simulink model "planta_PID_velocity"  (R2019b)
settings: Solver=ode23t  StartTime=0.0  StopTime=7  MaxStep=T  RelTol=1e-3  EnableMultiTasking=on
undefined symbols (not defined in the file): T
settings Model: Creator=fernandopassold  LastModifiedBy=fernandopassold
settings DataIOCC: LimitDataPoints=on  SaveFormat=Array  ReturnWorkspaceOutputs=off
settings OptimizationCC: LifeSpan=inf
settings DebuggingCC: SFUnexpectedBacktrackingDiag=warning  SFNoUnconditionalDefaultTransitionDiag=warning  SFExecutionAtInitializationDiag=none  ArithmeticOperatorsInVariantConditions=warning
settings HardwareCC: ProdBitPerPointer=32  ProdBitPerSizeT=32  ProdBitPerPtrDiffT=32  ProdLargestAtomicFloat=None  ProdIntDivRoundTo=Undefined  ProdEndianess=Unspecified  ProdWordSize=32  ProdHWDeviceType=32-bit Generic
settings ModelReferenceCC: PropagateSignalLabelsOutOfModel=off
settings SFSimCC: SimUseLocalCustomCode=off  CustomCodeUndefinedFunction=UseInterfaceOnly
settings RTWCC: RTWUseLocalCustomCode=off
settings CodeAppCC: StateflowObjectComments=on
settings GRTTargetCC: TargetLangStandard=C89/C90 (ANSI)  GeneratePreprocessorConditionals=Disable all
settings ConfigComp: CovMetricSettings=dw  CovHtmlReporting=on  CovSaveCumulativeToWorkspaceVar=on  CovSaveSingleToWorkspaceVar=on  CovExternalEMLEnable=off

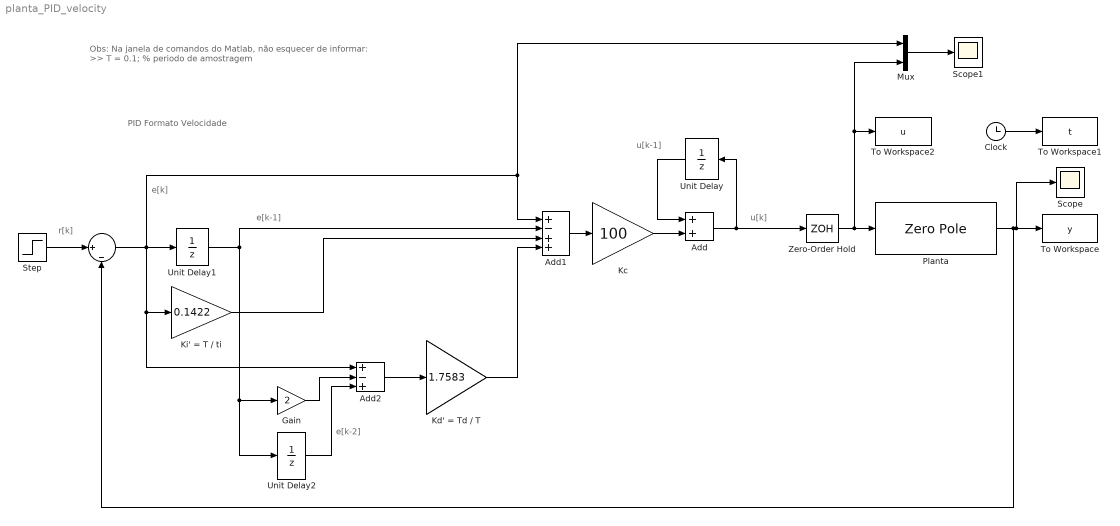
== system planta_PID_velocity ==
  note: Obs:
      | Na janela de comandos do Matlab, não esquecer de informar:
      | >> T = 0.1; % periodo de amostragem
  note: PID Formato Velocidade
  note: u[k-1]
  note: e[k-2]
  note: e[k-1]
  note: u[k]
  note: r[k]
  note: e[k]
  " " : Sum  Inputs=||+|-
  Add : Sum
  Add1 : Sum  Inputs=+|-|+|+
  Add2 : Sum  Inputs=+|-|+
  Clock : Clock
  Gain : Gain  Gain=2
  Kc : Gain  Gain=100
  Kd' = Td / T : Gain  Gain=1.7583
  Ki' = T / ti : Gain  Gain=0.1422
  Mux : Mux  Inputs=2
  Planta : ZeroPole  Zeros=[ ]  Poles="[-1  -2   -10]"
  Scope : Scope
  Scope1 : Scope
  Step : Step  Time=0  SampleTime=0
  To Workspace : ToWorkspace  VariableName=y  SaveFormat=Timeseries  SampleTime=-1
  To Workspace1 : ToWorkspace  VariableName=t  SampleTime=-1
  To Workspace2 : ToWorkspace  VariableName=u  SaveFormat=Timeseries  SampleTime=T
  Unit Delay : UnitDelay  SampleTime=T  HasFrameUpgradeWarning=on
  Unit Delay1 : UnitDelay  SampleTime=T  HasFrameUpgradeWarning=on
  Unit Delay2 : UnitDelay  SampleTime=T  HasFrameUpgradeWarning=on
  Zero-Order Hold : ZeroOrderHold  SampleTime=T
  wires:
  Step/1 -> " "/1
  Zero-Order Hold/1 -> Mux/2, To Workspace2/1, Planta/1
  Planta/1 -> Scope/1, To Workspace/1, " "/2
  Clock/1 -> To Workspace1/1
  Add/1 -> Unit Delay/1, Zero-Order Hold/1
  Unit Delay/1 -> Add/1
  Kc/1 -> Add/2
  Add1/1 -> Kc/1
  " "/1 -> Mux/1, Add1/1, Add2/1, Ki' = T / ti/1, Unit Delay1/1
  Unit Delay1/1 -> Gain/1, Unit Delay2/1, Add1/2
  Ki' = T / ti/1 -> Add1/3
  Add2/1 -> Kd' = Td / T/1
  Kd' = Td / T/1 -> Add1/4
  Gain/1 -> Add2/2
  Unit Delay2/1 -> Add2/3
  Mux/1 -> Scope1/1
